simulink model "project_6_PID_Only"  (R2020a)
settings: Solver=VariableStepAuto  StartTime=0.0  StopTime=10.0  MaxStep=0.01  RelTol=1e-3
values from neighbouring files (symbols this model uses):
  Kd = 50    [project_7m.m]    (also in project_8m.m = 207.6; project_9m.m = 2)
  Ki = 300    [project_7m.m]    (also in project_8m.m = 7398; project_9m.m = 4)
  Kp = 1    [project_6m.m]    (also in project_7m.m = 350; project_8m.m = 4433; project_9m.m = 8000)
settings Model: Creator=Matt  LastModifiedBy=Matt
settings DataIOCC: ReturnWorkspaceOutputs=off  TimeSaveName=time

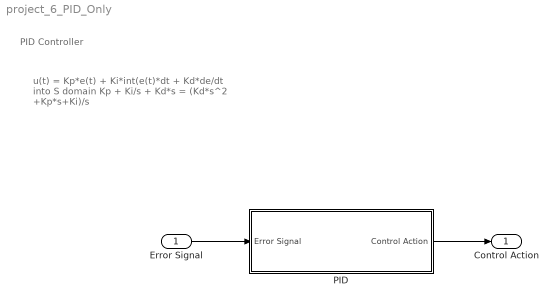
== system project_6_PID_Only ==
  note: u(t) = Kp*e(t) + Ki*int(e(t)*dt + Kd*de/dt
      | into S domain
      | Kp + Ki/s + Kd*s = (Kd*s^2 +Kp*s+Ki)/s
  note: PID Controller
  Error Signal : Inport
  PID : Subsystem
  Control Action : Outport
  wires:
  Error Signal/1 -> PID/1(Error Signal)
  PID/1(Control Action) -> Control Action/1

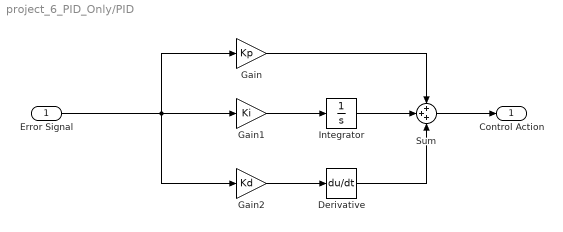
== system project_6_PID_Only/PID ==
  Error Signal : Inport
  Derivative : Derivative
  Gain : Gain  Gain=Kp
  Gain1 : Gain  Gain=Ki
  Gain2 : Gain  Gain=Kd
  Integrator : Integrator
  Sum : Sum  Inputs=+++
  Control Action : Outport
  wires:
  Derivative/1 -> Sum/3
  Error Signal/1 -> Gain2/1, Gain/1, Gain1/1
  Gain/1 -> Sum/1
  Sum/1 -> Control Action/1
  Integrator/1 -> Sum/2
  Gain1/1 -> Integrator/1
  Gain2/1 -> Derivative/1
